simulink model "rimless_wheel_sim_ver4"  (R2018b)
settings: Solver=ode8  StartTime=0.0  StopTime=10  FixedStep=1/1000  RelTol=1e-3
values from neighbouring files (symbols this model uses):
  teta0 = alfa-gama    (= -0.196349540849)    [parameters.m]
  teta1 = alfa+gama    (= 0.589048622548)    [parameters.m]
  w1 = sqrt(2*(g/l)*(1-cos(gama-alfa)))    [parameters.m]
  w2 = -sqrt(2*(g/l)*(1-cos(gama+alfa)))    [parameters.m]
libraries: simulink x1
settings Model: Creator=oguzh  LastModifiedBy=oguzh

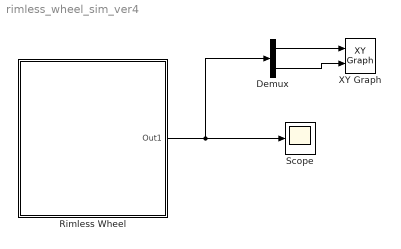
== system rimless_wheel_sim_ver4 ==
  Demux : Demux  Outputs=2
  Rimless Wheel : Subsystem  TreatAsAtomicUnit=on
      mask Display: image(imread('rimless_wheel.png'))
  Scope : Scope
  XY Graph : simulink/Sinks/XY Graph  xmin=-0.5  xmax=1  ymin=0  ymax=5  st=-1
  wires:
  Rimless Wheel/1(Out1) -> Demux/1, Scope/1
  Demux/1 -> XY Graph/1
  Demux/2 -> XY Graph/2

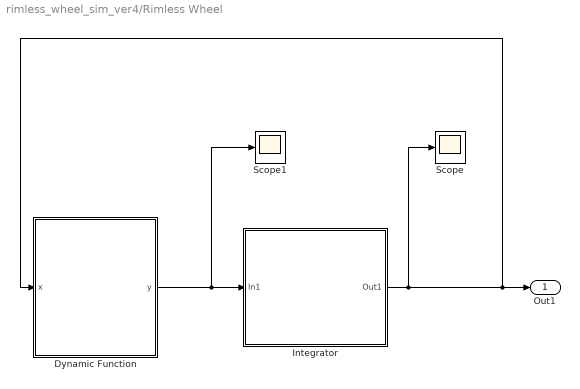
== system rimless_wheel_sim_ver4/Rimless Wheel ==
  Dynamic Function : MATLAB Function  TreatAsAtomicUnit=on
  Integrator : Subsystem
  Scope : Scope
  Scope1 : Scope
  Out1 : Outport
  wires:
  Dynamic Function/1(y) -> Scope1/1, Integrator/1(In1)
  Integrator/1(Out1) -> Out1/1, Dynamic Function/1(x), Scope/1

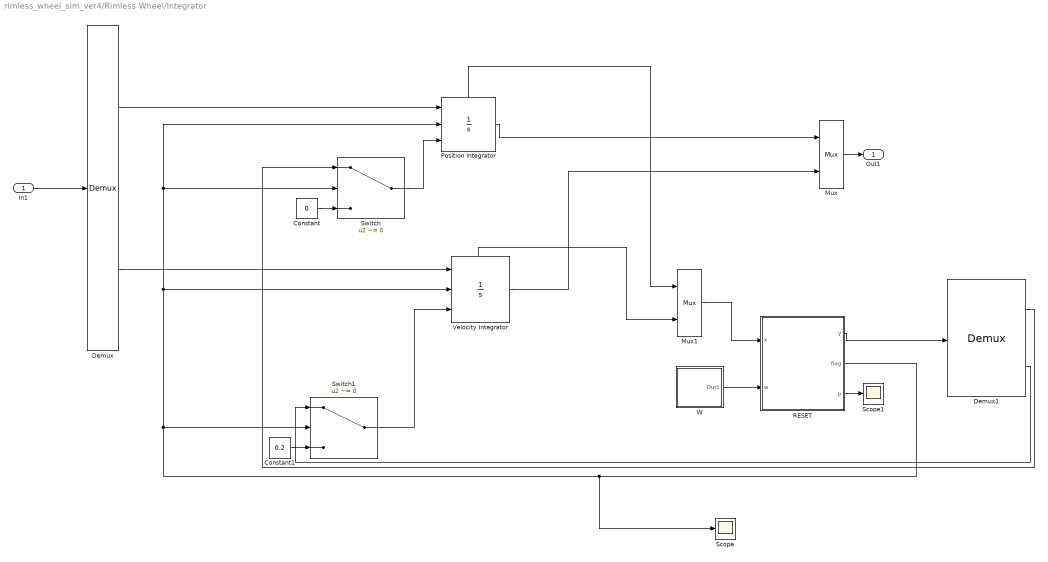
== system rimless_wheel_sim_ver4/Rimless Wheel/Integrator ==
  In1 : Inport
  Constant : Constant  Value=0
  Constant1 : Constant  Value=0.2
  Demux : Demux  Outputs=2
  Demux1 : Demux  Outputs=2
  Mux : Mux  Inputs=2
  Mux1 : Mux  Inputs=2
  Position Integrator : Integrator  ExternalReset=rising  InitialConditionSource=external  InitialCondition=0.002  UpperSaturationLimit=teta1  LowerSaturationLimit=teta0  ShowStatePort=on
  RESET : MATLAB Function  TreatAsAtomicUnit=on
  Scope : Scope
  Scope1 : Scope
  Switch : Switch  Criteria=u2 ~= 0  Threshold=1
  Switch1 : Switch  Criteria=u2 ~= 0  Threshold=1
  Velocity Integrator : Integrator  ExternalReset=rising  InitialConditionSource=external  ShowStatePort=on
  W : Subsystem
  Out1 : Outport
  wires:
  Demux/2 -> Velocity Integrator/1
  In1/1 -> Demux/1
  Demux/1 -> Position Integrator/1
  Mux/1 -> Out1/1
  W/1(Out1) -> RESET/2(w)
  RESET/1(y) -> Demux1/1
  RESET/2(flag) -> Scope/1, Switch1/2, Velocity Integrator/2, Switch/2, Position Integrator/2
  Constant/1 -> Switch/3
  Constant1/1 -> Switch1/3
  Demux1/1 -> Switch/1
  Demux1/2 -> Switch1/1
  Mux1/1 -> RESET/1(x)
  Velocity Integrator/State -> Mux1/2
  Position Integrator/State -> Mux1/1
  Switch/1 -> Position Integrator/3
  Switch1/1 -> Velocity Integrator/3
  Velocity Integrator/1 -> Mux/2
  Position Integrator/1 -> Mux/1
  RESET/3(p) -> Scope1/1

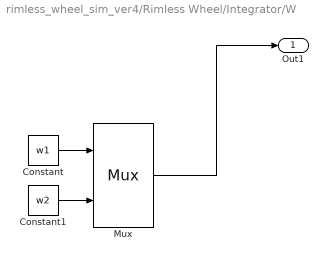
== system rimless_wheel_sim_ver4/Rimless Wheel/Integrator/W ==
  Constant : Constant  Value=w1
  Constant1 : Constant  Value=w2
  Mux : Mux  Inputs=2
  Out1 : Outport
  wires:
  Constant/1 -> Mux/1
  Constant1/1 -> Mux/2
  Mux/1 -> Out1/1

== matlab function rimless_wheel_sim_ver4/Rimless Wheel/Integrator/RESET ==
  data: x input; y output; w input; flag output; p output
function [y,flag,p] = fcn(x, w)
%% Parameters
l=0.5 ;         %length of a single scope
g=9.81  ;       %gravity
n=8    ;        %scope number
alfa= pi/16 ;    %slope angle
beta=2*pi/n ;     % angle of between the scopes
gama=beta/2;

teta0=alfa-gama;   % initial locomotion limit
teta1=alfa+gama;   % final locomotion limit

w1=w(1);
w2=w(2);

%% Reset Function
y=zeros(2,1);
flag=0;
p=0;
if x(1)>=teta1
                x(1)=teta0; 
                flag=1;
  
    if x(2)>w1
         x(2)=cos(beta)*sqrt(x(2)^2+4*(g/l)*sin(alfa)*sin(gama));
   p=1;
         

    elseif x(2)<w1 | x(2)>w2 == 1
          x(2)=-cos(beta)*x(2);
   p=2;
   
          
    elseif x(2)<w2
         x(2)=-cos(beta)*sqrt(x(2)^2-4*(g/l)*sin(alfa)*sin(gama));
   p=3;
  
         
    end
end
y=x;

== matlab function rimless_wheel_sim_ver4/Rimless Wheel/Dynamic Function ==
  data: x input; y output
function y = fcn(x)
%% Parameters
m=1  ;          %point mass
l=0.5 ;         %length of a single scope
g=9.81  ;       %gravity
n=8    ;        %scope number
alfa= pi/16 ;    %slope angle
beta=2*pi/n ;     % angle of between the scopes
gama=beta/2;

teta0=alfa-gama;   % initial locomotion limit
teta1=alfa+gama;   % final locomotion limit

%% Initialization
q=0;
dq=0;
fx=zeros(2,1);

q=x(1);
dq=x(2);



%% Dynamics
fx=[dq
    (g/l)*sin(q)];

y = fx;
